simulink model "dc_gain"  (R2018b)
settings: Solver=ode8  StartTime=0.0  StopTime=10  FixedStep=0.001  RelTol=1e-3
model workspace (MAT data in the model file):
  A = Simulink.Parameter
  A.Value = 1
  A.DataType = 'auto'
  A.DocUnits = 'm^2'
  A.Dimensions = [1 1]
  K = Simulink.Parameter
  K.Value = Simulink.data.Expression
  K.Value.ExpressionString = "1/k1"
  K.DataType = 'auto'
  K.DocUnits = 's/m^2'
  K.Dimensions = -1
  h0 = Simulink.Parameter
  h0.Value = 0
  h0.DataType = 'auto'
  h0.DocUnits = 'm'
  h0.Dimensions = [1 1]
  k1 = Simulink.Parameter
  k1.Value = 10
  k1.DataType = 'auto'
  k1.DocUnits = 'm^2/s'
  k1.Dimensions = [1 1]
  qin = Simulink.Parameter
  qin.Value = 0.4
  qin.DataType = 'auto'
  qin.DocUnits = 'm^3/s'
  qin.Dimensions = [1 1]
  tau = Simulink.Parameter
  tau.Value = Simulink.data.Expression
  tau.Value.ExpressionString = "A/k1"
  tau.DataType = 'auto'
  tau.DocUnits = 's'
  tau.Dimensions = -1
settings Model: OrderedModelArguments=off  Creator=waleed.elbadry  LastModifiedBy=waleed.elbadry
settings SolverCC: MaxConsecutiveZCs=100000
settings CodeAppCC: StateflowObjectComments=on

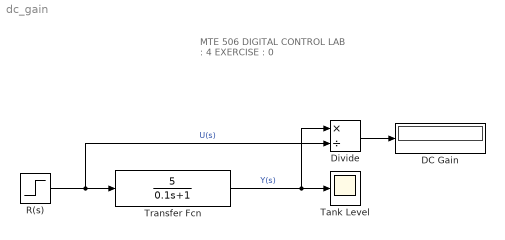
== system dc_gain ==
  note: MTE 506 DIGITAL CONTROL
      | LAB : 4
      | EXERCISE : 0
  DC Gain : Display
  Divide : Product  Inputs=*/
  R(s) : Step  Time=0  SampleTime=0
  Tank Level : Scope
  Transfer Fcn : TransferFcn  Numerator=[5]  Denominator=[0.1 1]
  wires:
  Transfer Fcn/1 -> Divide/1, Tank Level/1  "Y(s)"
  R(s)/1 -> Divide/2, Transfer Fcn/1  "U(s)"
  Divide/1 -> DC Gain/1
